simulink library "block_library"  (R2021b)
settings: Solver=VariableStepAuto  StartTime=0.0  StopTime=10.0  RelTol=1e-3
values from neighbouring files (symbols this model uses):
  d = param(17)    [get_full_state.m]
  gravity = [param(6), param(7),param(8)]    [get_ac_forces_moments.m]
  k_line = param(18)    [get_full_state.m]
  q = 0.5*rho*V_a^2    [aircraft_sizing_optimization.m]    (also in get_ac_forces_moments.m = state(11))
  r = state(12)    [get_ac_forces_moments.m]
  rho = rho_0*exp(-h/h1)    [aircraft_sizing_optimization.m]    (also in get_ac_forces_moments.m = param(2); get_simple_state.m = const(7))
undefined symbols (not defined in the file or in its folder): c, F, InitTheta, InitThetaDot, k_damp, k_pitch, k_roll, Light, magnitude, MIL, moi, motor_kt, motor_moi, state1, WindVelocity
libraries: aerolibwind2 x3, aerolibasang x2, vrlib x2, shared6dof x1, sharedtransform x1, sharedutil x1
settings Model: Creator=austm  LastModifiedBy=austm

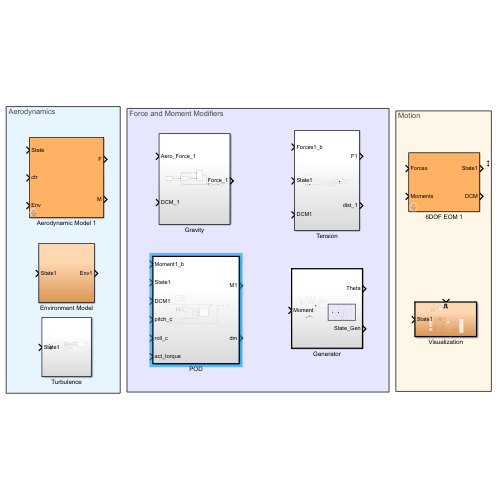
[thumbnail: Simulink's stored preview of the top-level diagram]
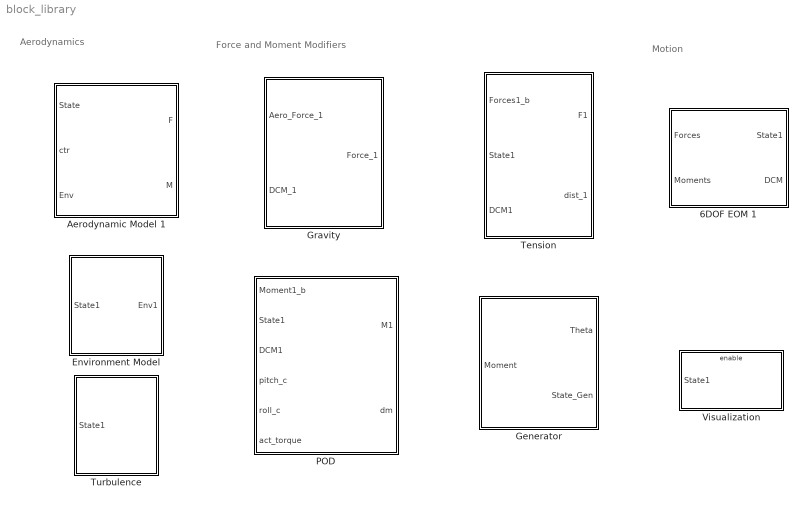
== system block_library ==
  note: Motion
  note: Force and Moment Modifiers
  note: Aerodynamics
  6DOF EOM 1 : Subsystem  VariantControl=eom3DOF  mask{XYZ=[0, 0, 0], uvw=[0, 0, 0], rpy=[0, 0, 0], pqr=[0, 0, 0], m=1, I=[1, 0, 0; 0, 1, 0; 0, 0, 1]}
      mask prompts: XYZ "Initial position in inertial axes [Xe,Ye,Ze]"; uvw "Initial velocity in body axes [U,v,w]"; rpy "Initial Euler orientation [roll, pitch, yaw]"; pqr "Initial body rotation rates [p,q,r]"; m "Initial mass"; I "Inertia"
  Aerodynamic Model 1 : Subsystem  VariantControl=aeroCONST  mask{CG=[0, 0, 0], CP=[0, 0, 0]}
      mask prompts: CG "Center of Gravity"; CP "Center of Pressure"
  Environment Model : Subsystem  VariantControl=aeroCONST
  Generator : Subsystem  TreatAsAtomicUnit=on
  Gravity : Subsystem
  POD : Subsystem  TreatAsAtomicUnit=on
  Tension : Subsystem
  Turbulence : Subsystem
  Visualization : Subsystem

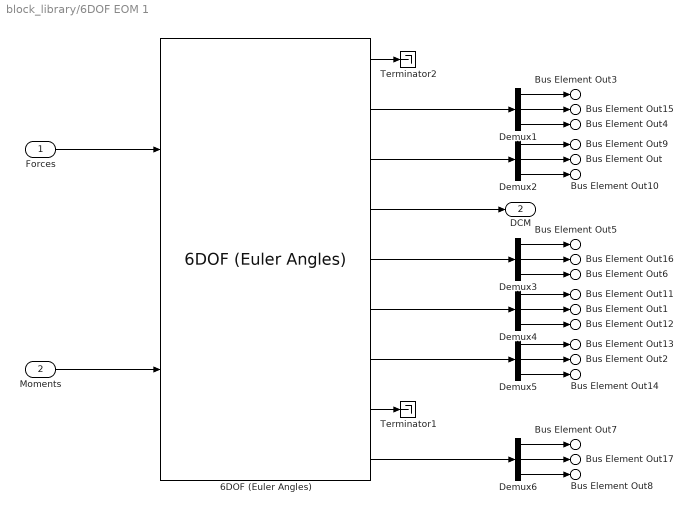
== system block_library/6DOF EOM 1 ==
  Forces : Inport
  Moments : Inport  Port=2
  6DOF (Euler Angles) : shared6dof/6DOF (Euler Angles)  units=Metric (MKS)  mtype=Fixed  rep=Euler Angles  xme_0=XYZ  Vm_0=uvw  eul_0=rpy  pm_0=pqr  mass_0=m  mass_e=0.5  mass_f=2.0  inertia=I  inertia_e=eye(3)  inertia_f=2*eye(3)  k_quat=1.0  vre_flag=on  abi_flag=on  aMode=0  xme_statename={'Xe', 'Ye', 'Ze'}  Vm_statename={'U', 'V', 'W'}  eul_statename={'phi', 'theta', 'psi'}  quat_statename={'qr', 'qi', 'qj','qk'}  pm_statename={'p', 'q', 'r'}  mass_statename=''
      settings: SourceProductBaseCode=AE,PW,DR,MT,UV,VE
  Demux{1..6} (6 alike) : Demux  Outputs=3
  Terminator1 : Terminator
  Terminator2 : Terminator
  Bus Element Out3 : Outport  VectorParamsAs1DForOutWhenUnconnected=off  PortName=State1  Element=Xe
  Bus Element Out4 : Outport  VectorParamsAs1DForOutWhenUnconnected=off  PortName=State1  Element=Ze
  Bus Element Out : Outport  VectorParamsAs1DForOutWhenUnconnected=off  PortName=State1  Element=theta
  Bus Element Out5 : Outport  VectorParamsAs1DForOutWhenUnconnected=off  PortName=State1  Element=u
  Bus Element Out6 : Outport  VectorParamsAs1DForOutWhenUnconnected=off  PortName=State1  Element=w
  Bus Element Out1 : Outport  VectorParamsAs1DForOutWhenUnconnected=off  PortName=State1  Element=q
  Bus Element Out2 : Outport  VectorParamsAs1DForOutWhenUnconnected=off  PortName=State1  Element=q_dot
  Bus Element Out7 : Outport  VectorParamsAs1DForOutWhenUnconnected=off  PortName=State1  Element=Axe
  Bus Element Out8 : Outport  VectorParamsAs1DForOutWhenUnconnected=off  PortName=State1  Element=Aze
  Bus Element Out15 : Outport  VectorParamsAs1DForOutWhenUnconnected=off  PortName=State1  Element=Ye
  Bus Element Out9 : Outport  VectorParamsAs1DForOutWhenUnconnected=off  PortName=State1  Element=phi
  Bus Element Out10 : Outport  VectorParamsAs1DForOutWhenUnconnected=off  PortName=State1  Element=psi
  Bus Element Out16 : Outport  VectorParamsAs1DForOutWhenUnconnected=off  PortName=State1  Element=v
  Bus Element Out11 : Outport  VectorParamsAs1DForOutWhenUnconnected=off  PortName=State1  Element=p
  Bus Element Out12 : Outport  VectorParamsAs1DForOutWhenUnconnected=off  PortName=State1  Element=r
  Bus Element Out13 : Outport  VectorParamsAs1DForOutWhenUnconnected=off  PortName=State1  Element=p_dot
  Bus Element Out14 : Outport  VectorParamsAs1DForOutWhenUnconnected=off  PortName=State1  Element=r_dot
  Bus Element Out17 : Outport  VectorParamsAs1DForOutWhenUnconnected=off  PortName=State1  Element=Aye
  DCM : Outport  Port=2
  wires:
  6DOF (Euler Angles)/2 -> Demux1/1
  6DOF (Euler Angles)/4 -> DCM/1
  6DOF (Euler Angles)/1 -> Terminator2/1
  Demux6/2 -> Bus Element Out17/1
  Demux6/3 -> Bus Element Out8/1
  Demux6/1 -> Bus Element Out7/1
  6DOF (Euler Angles)/9 -> Demux6/1
  6DOF (Euler Angles)/7 -> Demux5/1
  Demux5/3 -> Bus Element Out14/1
  Demux5/2 -> Bus Element Out2/1
  Demux5/1 -> Bus Element Out13/1
  6DOF (Euler Angles)/6 -> Demux4/1
  Demux4/3 -> Bus Element Out12/1
  Demux4/2 -> Bus Element Out1/1
  Demux4/1 -> Bus Element Out11/1
  Demux3/3 -> Bus Element Out6/1
  Demux3/2 -> Bus Element Out16/1
  Demux3/1 -> Bus Element Out5/1
  6DOF (Euler Angles)/5 -> Demux3/1
  Demux2/3 -> Bus Element Out10/1
  Demux2/2 -> Bus Element Out/1
  Demux2/1 -> Bus Element Out9/1
  Demux1/1 -> Bus Element Out3/1
  Demux1/3 -> Bus Element Out4/1
  Demux1/2 -> Bus Element Out15/1
  6DOF (Euler Angles)/3 -> Demux2/1
  Moments/1 -> 6DOF (Euler Angles)/2
  Forces/1 -> 6DOF (Euler Angles)/1
  6DOF (Euler Angles)/8 -> Terminator1/1

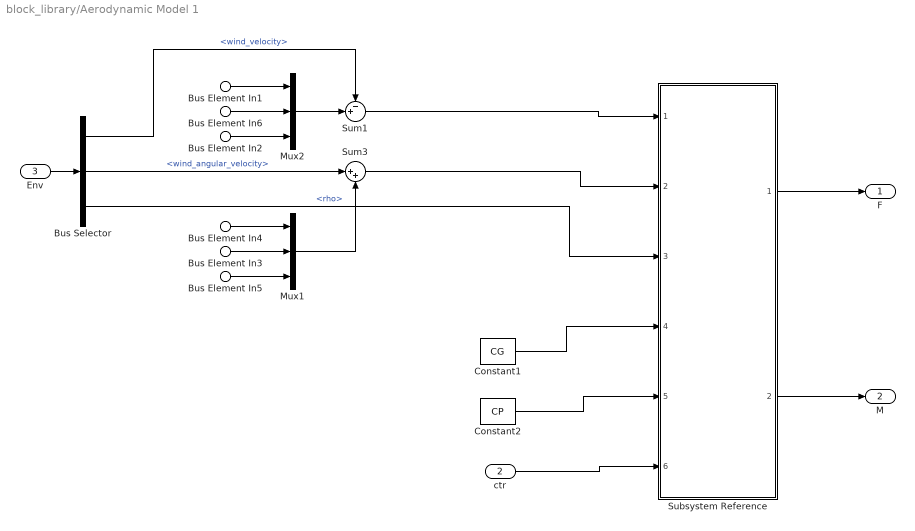
== system block_library/Aerodynamic Model 1 ==
  Bus Element In1 : Inport  PortName=State  Element=u
  Bus Element In2 : Inport  PortName=State  Element=w
  Bus Element In3 : Inport  PortName=State  Element=q
  Bus Element In6 : Inport  PortName=State  Element=v
  Bus Element In4 : Inport  PortName=State  Element=p
  Bus Element In5 : Inport  PortName=State  Element=r
  ctr : Inport  Port=2
  Env : Inport  Port=3
  Bus Selector : BusSelector  OutputSignals=wind_velocity,wind_angular_velocity,rho
  Constant1 : Constant  Value=CG
  Constant2 : Constant  Value=CP
  Mux1 : Mux  Inputs=3
  Mux2 : Mux  Inputs=3
  Subsystem Reference : Subsystem  ReferencedSubsystem=Aerodynamics
  Sum1 : Sum  Inputs=-+|  InputSameDT=on  SaturateOnIntegerOverflow=on  OutDataTypeStr=Inherit: Same as first input
  Sum3 : Sum  Inputs=|++  InputSameDT=on  SaturateOnIntegerOverflow=on  OutDataTypeStr=Inherit: Same as first input
  F : Outport  Unit=N  VectorParamsAs1DForOutWhenUnconnected=off
  M : Outport  Port=2  Unit=N*m  VectorParamsAs1DForOutWhenUnconnected=off
  wires:
  Bus Selector/1 -> Sum1/1  "<wind_velocity>"
  Mux2/1 -> Sum1/2
  Mux1/1 -> Sum3/2
  Bus Selector/2 -> Sum3/1  "<wind_angular_velocity>"
  Bus Element In5/1 -> Mux1/3
  Bus Element In3/1 -> Mux1/2
  Bus Element In4/1 -> Mux1/1
  Bus Element In1/1 -> Mux2/1
  Bus Element In6/1 -> Mux2/2
  Bus Element In2/1 -> Mux2/3
  Sum1/1 -> Subsystem Reference/1
  Sum3/1 -> Subsystem Reference/2
  Bus Selector/3 -> Subsystem Reference/3  "<rho>"
  Constant1/1 -> Subsystem Reference/4
  Constant2/1 -> Subsystem Reference/5
  Subsystem Reference/1 -> F/1
  Subsystem Reference/2 -> M/1
  ctr/1 -> Subsystem Reference/6
  Env/1 -> Bus Selector/1

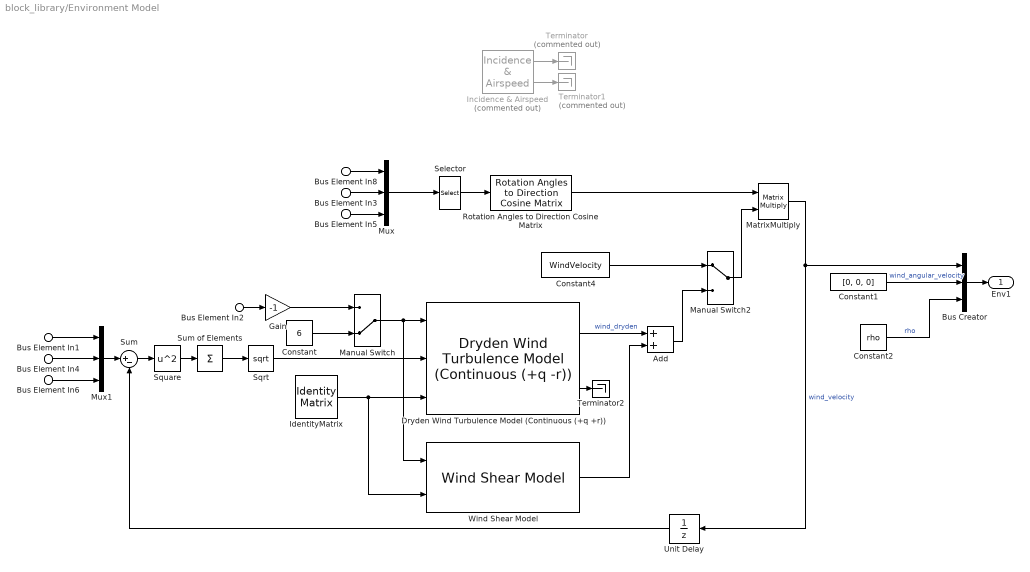
== system block_library/Environment Model ==
  Bus Element In3 : Inport  PortName=State1  Element=theta
  Bus Element In8 : Inport  PortName=State1  Element=phi
  Bus Element In5 : Inport  PortName=State1  Element=psi
  Bus Element In1 : Inport  PortName=State1  Element=u
  Bus Element In2 : Inport  PortName=State1  Element=Ze
  Bus Element In4 : Inport  PortName=State1  Element=v
  Bus Element In6 : Inport  PortName=State1  Element=w
  Add : Sum
  Bus Creator : BusCreator  Inputs=3
  Constant : Constant  Value=6
  Constant1 : Constant  Value=[0, 0, 0]
  Constant2 : Constant  Value=rho
  Constant4 : Constant  Value=WindVelocity
  Dryden Wind Turbulence Model (Continuous (+q +r)) : aerolibwind2/Dryden Wind Turbulence Model  (Continuous (+q -r))  units=Metric (MKS)  spec=MIL-F-8785C  model=Continuous Dryden (+q +r)  W20=WindVelocity(1)  Wdeg=0  TurbProb=10^-2 - Light  L_high=533.4  Wingspan=3  ts=0.1  Seed=[23341 23342 23343 23344]  T_on=on
  Gain : Gain  Gain=-1
  IdentityMatrix : IdentityMatrix  OutputDimensions=3
  Incidence & Airspeed : aerolibasang/Incidence  & Airspeed  Commented=on
      settings: SourceProductBaseCode=AE
  Manual Switch : ManualSwitch  CurrentSetting=0
  Manual Switch2 : ManualSwitch
  MatrixMultiply : Product  Multiplication=Matrix(*)
  Mux : Mux  Inputs=3
  Mux1 : Mux  Inputs=3
  Rotation Angles to Direction Cosine Matrix : sharedtransform/Rotation Angles to Direction Cosine Matrix  rotationOrder=ZYX  aMode=aMode
      settings: SourceProductBaseCode=AE,PW,DR,MT,UV,VE
  Selector : Selector  InputPortWidth=3  IndexOptions=Index vector (dialog)  Indices=[3 2 1]  OutputSizes=1
  Sqrt : Sqrt  SaturateOnIntegerOverflow=on
  Square : Math  Operator=square  SaturateOnIntegerOverflow=on
  Sum : Sum  Inputs=|+-
  Sum of Elements : Sum  Inputs=+
  Terminator : Terminator  Commented=on
  Terminator1 : Terminator  Commented=on
  Terminator2 : Terminator
  Unit Delay : UnitDelay  InitialCondition=norm(WindVelocity)  SampleTime=-1  HasFrameUpgradeWarning=on
  Wind Shear Model : aerolibwind2/Wind Shear Model  units=Metric (MKS)  phase=Category C - Terminal Flight Phase  W_20=norm(WindVelocity)  Wdeg=atan2d(WindVelocity(2), WindVelocity(1))+180
  Env1 : Outport
  wires:
  Constant1/1 -> Bus Creator/2  "wind_angular_velocity"
  Dryden Wind Turbulence Model (Continuous (+q +r))/1 -> Add/1  "wind_dryden"
  Rotation Angles to Direction Cosine Matrix/1 -> MatrixMultiply/1
  Bus Element In5/1 -> Mux/3
  Mux/1 -> Selector/1
  Incidence & Airspeed/2 -> Terminator1/1
  Incidence & Airspeed/1 -> Terminator/1
  Constant2/1 -> Bus Creator/3  "rho"
  Bus Element In8/1 -> Mux/1
  Bus Element In3/1 -> Mux/2
  MatrixMultiply/1 -> Bus Creator/1, Unit Delay/1  "wind_velocity"
  Selector/1 -> Rotation Angles to Direction Cosine Matrix/1
  Bus Creator/1 -> Env1/1
  Manual Switch/1 -> Dryden Wind Turbulence Model (Continuous (+q +r))/1, Wind Shear Model/1
  Bus Element In1/1 -> Mux1/1
  IdentityMatrix/1 -> Wind Shear Model/2, Dryden Wind Turbulence Model (Continuous (+q +r))/3
  Dryden Wind Turbulence Model (Continuous (+q +r))/2 -> Terminator2/1
  Add/1 -> Manual Switch2/2
  Bus Element In2/1 -> Gain/1
  Bus Element In4/1 -> Mux1/2
  Bus Element In6/1 -> Mux1/3
  Mux1/1 -> Sum/1
  Sum/1 -> Square/1
  Square/1 -> Sum of Elements/1
  Sum of Elements/1 -> Sqrt/1
  Sqrt/1 -> Dryden Wind Turbulence Model (Continuous (+q +r))/2
  Constant/1 -> Manual Switch/2
  Gain/1 -> Manual Switch/1
  Unit Delay/1 -> Sum/2
  Wind Shear Model/1 -> Add/2
  Constant4/1 -> Manual Switch2/1
  Manual Switch2/1 -> MatrixMultiply/2

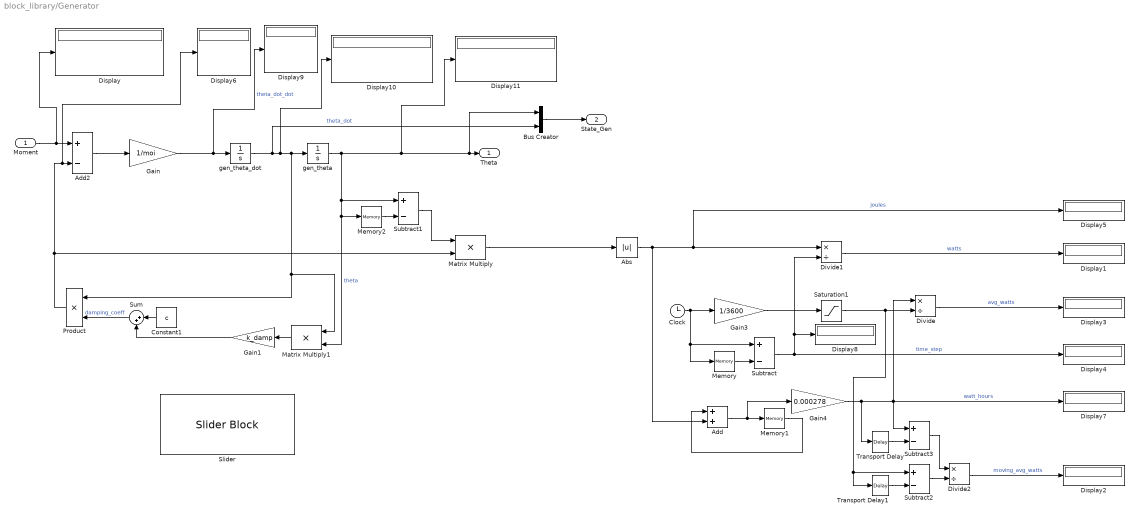
== system block_library/Generator ==
  Moment : Inport
  Abs : Abs
  Add : Sum
  Add2 : Sum  Inputs=+-
  Bus Creator : BusCreator  Inputs=2
  Clock : Clock
  Constant1 : Constant  Value=c
  Display{,1..11} (12 alike) : Display
      Display settings: Format=long_e  Decimation=6
      Display10 settings: Format=long_e
      Display11 settings: Format=long_e
  Divide : Product  Inputs=*/
  Divide1 : Product  Inputs=*/
  Divide2 : Product  Inputs=*/
  Gain : Gain  Gain=1/moi
  Gain1 : Gain  Gain=k_damp
  Gain3 : Gain  Gain=1/3600
  Gain4 : Gain  Gain=0.000278
  Matrix Multiply : Product
  Matrix Multiply1 : Product
  Memory : Memory  InitialCondition=-.001
  Memory1 : Memory
  Memory2 : Memory
  Product : Product
  Saturation1 : Saturate  UpperLimit=inf  LowerLimit=0.00001
  Slider : SliderBlock  ScaleMax=500
  Subtract{,1..3} (4 alike) : Sum  Inputs=+-
  Sum : Sum  Inputs=|++
  Transport Delay : TransportDelay  DelayTime=30  BufferSize=10240
  Transport Delay1 : TransportDelay  DelayTime=30  BufferSize=10240
  gen_theta : Integrator  InitialCondition=InitTheta
  gen_theta_dot : Integrator  InitialCondition=InitThetaDot
  Theta : Outport
  State_Gen : Outport  Port=2
  wires:
  Bus Creator/1 -> State_Gen/1
  Saturation1/1 -> Transport Delay1/1, Subtract2/1, Divide/2
  Divide2/1 -> Display2/1  "moving_avg_watts"
  Subtract3/1 -> Divide2/1
  Transport Delay/1 -> Subtract3/2
  Subtract2/1 -> Divide2/2
  Transport Delay1/1 -> Subtract2/2
  Gain1/1 -> Sum/2
  Sum/1 -> Product/2  "damping_coeff"
  Constant1/1 -> Sum/1
  Memory2/1 -> Subtract1/2
  Gain4/1 -> Transport Delay/1, Divide/1, Subtract3/1, Display7/1  "watt_hours"
  Memory1/1 -> Add/1
  Add/1 -> Gain4/1, Memory1/1
  Matrix Multiply/1 -> Abs/1
  Divide1/1 -> Display1/1  "watts"
  Subtract/1 -> Display4/1, Display8/1, Divide1/2  "time_step"
  Memory/1 -> Subtract/2
  Divide/1 -> Display3/1  "avg_watts"
  Gain3/1 -> Saturation1/1
  Clock/1 -> Gain3/1, Subtract/1, Memory/1
  Product/1 -> Display6/1, Add2/2, Matrix Multiply/2
  Matrix Multiply1/1 -> Gain1/1
  Abs/1 -> Add/2, Divide1/1, Display5/1  "joules"
  Subtract1/1 -> Matrix Multiply/1
  gen_theta/1 -> Subtract1/1, Memory2/1, Matrix Multiply1/2, Display11/1, Bus Creator/1, Theta/1  "theta"
  gen_theta_dot/1 -> Display10/1, gen_theta/1, Matrix Multiply1/1, Product/1, Bus Creator/2  "theta_dot"
  Gain/1 -> Display9/1, gen_theta_dot/1  "theta_dot_dot"
  Add2/1 -> Gain/1
  Moment/1 -> Add2/1, Display/1

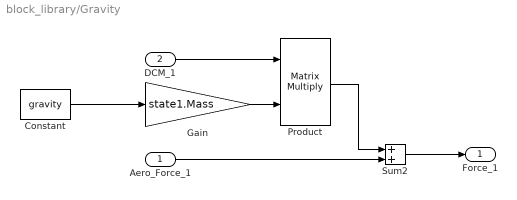
== system block_library/Gravity ==
  Aero_Force_1 : Inport
  DCM_1 : Inport  Port=2
  Constant : Constant  Value=gravity
  Gain : Gain  Gain=state1.Mass
  Product : Product  Multiplication=Matrix(*)
  Sum2 : Sum  InputSameDT=on  SaturateOnIntegerOverflow=on  OutDataTypeStr=Inherit: Same as first input
  Force_1 : Outport
  wires:
  Gain/1 -> Product/2
  Product/1 -> Sum2/1
  DCM_1/1 -> Product/1
  Aero_Force_1/1 -> Sum2/2
  Sum2/1 -> Force_1/1
  Constant/1 -> Gain/1

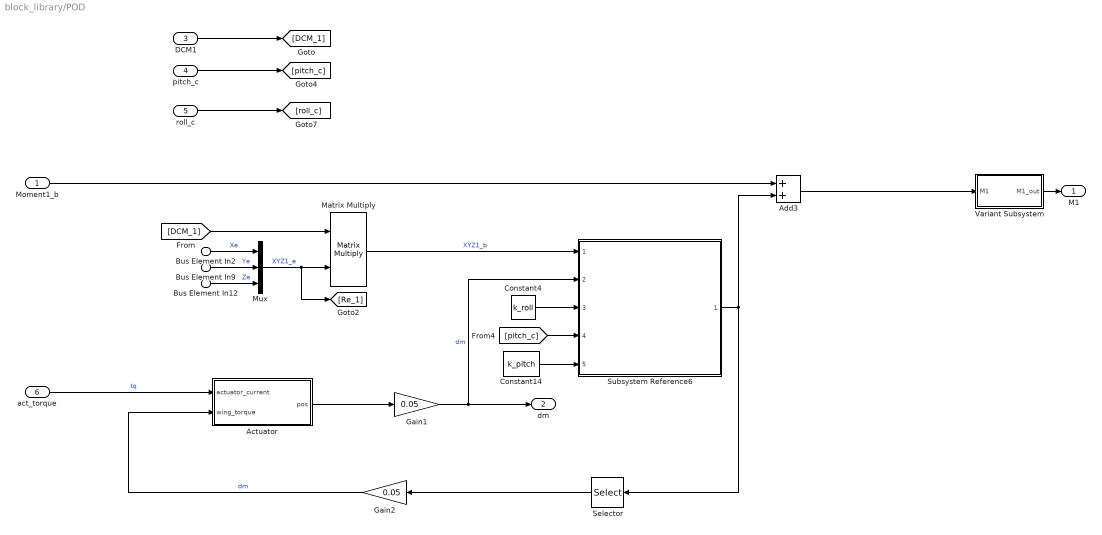
== system block_library/POD ==
  Moment1_b : Inport
  Bus Element In12 : Inport  Port=2  PortName=State1  Element=Ze
  Bus Element In2 : Inport  Port=2  PortName=State1  Element=Xe
  Bus Element In9 : Inport  Port=2  PortName=State1  Element=Ye
  DCM1 : Inport  Port=3
  pitch_c : Inport  Port=4
  roll_c : Inport  Port=5
  act_torque : Inport  Port=6
  Actuator : Subsystem
  Add3 : Sum
  Constant14 : Constant  Value=k_pitch
  Constant4 : Constant  Value=k_roll
  Gain1 : Gain  Gain=0.05
  Gain2 : Gain  Gain=0.05
  Matrix Multiply : Product  Multiplication=Matrix(*)
  Mux : Mux  Inputs=3
  Selector : Selector  InputPortWidth=3  IndexOptions=Index vector (dialog)  Indices=1  OutputSizes=1
  Subsystem Reference6 : Subsystem  ReferencedSubsystem=control_moments
  Variant Subsystem : Subsystem  Variant=on
  M1 : Outport
  dm : Outport  Port=2
  wires:
  Constant14/1 -> Subsystem Reference6/5
  [pitch_c] -> Subsystem Reference6/4
  Constant4/1 -> Subsystem Reference6/3
  Subsystem Reference6/1 -> Add3/2, Selector/1
  Matrix Multiply/1 -> Subsystem Reference6/1  "XYZ1_b"
  Moment1_b/1 -> Add3/1
  DCM1/1 -> [DCM_1]
  Bus Element In2/1 -> Mux/1  "Xe"
  Bus Element In12/1 -> Mux/3  "Ze"
  Bus Element In9/1 -> Mux/2  "Ye"
  Mux/1 -> Matrix Multiply/2, [Re_1]  "XYZ1_e"
  [DCM_1] -> Matrix Multiply/1
  Variant Subsystem/1(M1_out) -> M1/1
  roll_c/1 -> [roll_c]
  pitch_c/1 -> [pitch_c]
  Add3/1 -> Variant Subsystem/1(M1)
  Gain1/1 -> Subsystem Reference6/2, dm/1  "dm"
  act_torque/1 -> Actuator/1(actuator_current)  "tq"
  Selector/1 -> Gain2/1
  Actuator/1(pos) -> Gain1/1
  Gain2/1 -> Actuator/2(wing_torque)  "dm"

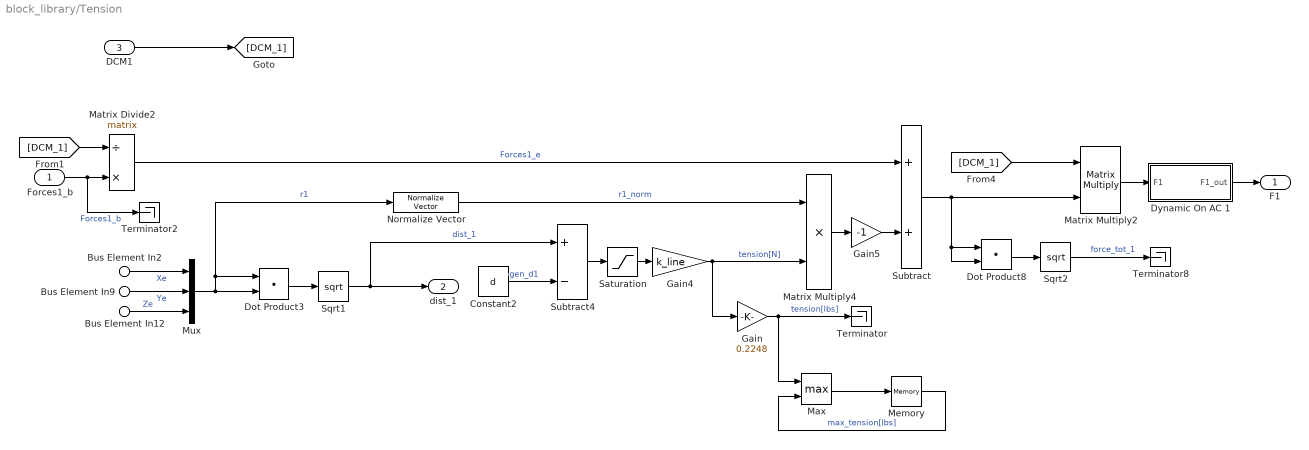
== system block_library/Tension ==
  Forces1_b : Inport
  Bus Element In12 : Inport  Port=2  PortName=State1  Element=Ze
  Bus Element In2 : Inport  Port=2  PortName=State1  Element=Xe
  Bus Element In9 : Inport  Port=2  PortName=State1  Element=Ye
  DCM1 : Inport  Port=3
  Constant2 : Constant  Value=d
  Dot Product3 : DotProduct  InputSameDT=on  OutDataTypeStr=Inherit: Inherit via internal rule
  Dot Product8 : DotProduct  InputSameDT=on  OutDataTypeStr=Inherit: Inherit via internal rule
  Dynamic On AC 1 : Subsystem  Variant=on
  Gain : Gain  Gain=0.2248
  Gain4 : Gain  Gain=k_line
  Gain5 : Gain  Gain=-1
  Matrix Divide2 : Product  Inputs=/*  Multiplication=Matrix(*)
  Matrix Multiply2 : Product  Multiplication=Matrix(*)
  Matrix Multiply4 : Product
  Max : MinMax  Function=max  Inputs=2
  Memory : Memory
  Mux : Mux  Inputs=3
  Normalize Vector : vrlib/Utilities/Normalize Vector  maxzero=0
  Saturation : Saturate  UpperLimit=inf  LowerLimit=0
  Sqrt1 : Sqrt  SaturateOnIntegerOverflow=on
  Sqrt2 : Sqrt  SaturateOnIntegerOverflow=on
  Subtract : Sum
  Subtract4 : Sum  Inputs=+-
  Terminator : Terminator
  Terminator2 : Terminator
  Terminator8 : Terminator
  F1 : Outport  Unit=N  VectorParamsAs1DForOutWhenUnconnected=off
  dist_1 : Outport  Port=2
  wires:
  Bus Element In2/1 -> Mux/1  "Xe"
  Bus Element In9/1 -> Mux/2  "Ye"
  Bus Element In12/1 -> Mux/3  "Ze"
  DCM1/1 -> [DCM_1]
  [DCM_1] -> Matrix Divide2/1
  Matrix Multiply2/1 -> Dynamic On AC 1/1(F1)
  [DCM_1] -> Matrix Multiply2/1
  Forces1_b/1 -> Terminator2/1, Matrix Divide2/2  "Forces1_b"
  Subtract/1 -> Dot Product8/2, Dot Product8/1, Matrix Multiply2/2
  Mux/1 -> Normalize Vector/1, Dot Product3/1, Dot Product3/2  "r1"
  Dot Product3/1 -> Sqrt1/1
  Sqrt1/1 -> Subtract4/1, dist_1/1  "dist_1"
  Gain5/1 -> Subtract/2
  Dynamic On AC 1/1(F1_out) -> F1/1
  Matrix Divide2/1 -> Subtract/1  "Forces1_e"
  Sqrt2/1 -> Terminator8/1  "force_tot_1"
  Dot Product8/1 -> Sqrt2/1
  Normalize Vector/1 -> Matrix Multiply4/1  "r1_norm"
  Gain4/1 -> Gain/1, Matrix Multiply4/2  "tension[N]"
  Constant2/1 -> Subtract4/2  "gen_d1"
  Matrix Multiply4/1 -> Gain5/1
  Subtract4/1 -> Saturation/1
  Saturation/1 -> Gain4/1
  Gain/1 -> Max/1, Terminator/1  "tension[lbs]"
  Max/1 -> Memory/1
  Memory/1 -> Max/2  "max_tension[lbs]"

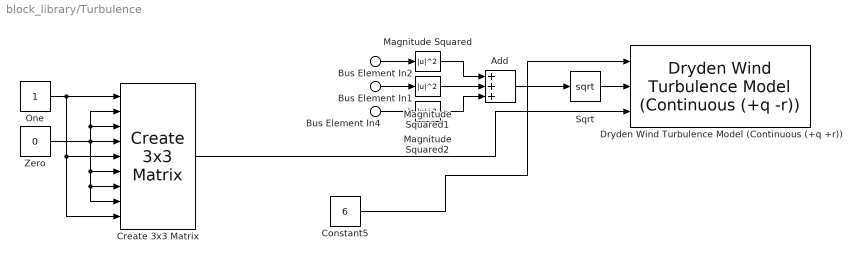
== system block_library/Turbulence ==
  Bus Element In2 : Inport  PortName=State1  Element=u
  Bus Element In1 : Inport  PortName=State1  Element=v
  Bus Element In4 : Inport  PortName=State1  Element=w
  Add : Sum  Inputs=+++
  Constant5 : Constant  Value=6
  Create 3x3 Matrix : sharedutil/Create 3x3 Matrix  aMode=aMode
      settings: SourceProductBaseCode=AE,PW,DR,MT,UV,VE
  Dryden Wind Turbulence Model (Continuous (+q +r)) : aerolibwind2/Dryden Wind Turbulence Model  (Continuous (+q -r))  units=Metric (MKS)  spec=MIL-F-8785C  model=Continuous Dryden (+q +r)  W20=3  Wdeg=180  TurbProb=10^-2 - Light  L_high=533.4  Wingspan=3  ts=0.1  Seed=[23341 23342 23343 23344]  T_on=off
  Magnitude Squared : Math  Operator=magnitude^2  SaturateOnIntegerOverflow=on
  Magnitude Squared1 : Math  Operator=magnitude^2  SaturateOnIntegerOverflow=on
  Magnitude Squared2 : Math  Operator=magnitude^2  SaturateOnIntegerOverflow=on
  One : Constant  OutDataTypeStr=Inherit: Inherit via back propagation
  Sqrt : Sqrt  SaturateOnIntegerOverflow=on
  Zero : Constant  Value=0  OutDataTypeStr=Inherit: Inherit via back propagation
  wires:
  Magnitude Squared2/1 -> Add/3
  Magnitude Squared/1 -> Add/1
  Constant5/1 -> Dryden Wind Turbulence Model (Continuous (+q +r))/1
  Magnitude Squared1/1 -> Add/2
  Zero/1 -> Create 3x3 Matrix/8, Create 3x3 Matrix/7, Create 3x3 Matrix/6, Create 3x3 Matrix/3, Create 3x3 Matrix/2, Create 3x3 Matrix/4
  Bus Element In4/1 -> Magnitude Squared2/1
  Bus Element In2/1 -> Magnitude Squared/1
  One/1 -> Create 3x3 Matrix/9, Create 3x3 Matrix/5, Create 3x3 Matrix/1
  Sqrt/1 -> Dryden Wind Turbulence Model (Continuous (+q +r))/2
  Add/1 -> Sqrt/1
  Bus Element In1/1 -> Magnitude Squared1/1
  Create 3x3 Matrix/1 -> Dryden Wind Turbulence Model (Continuous (+q +r))/3

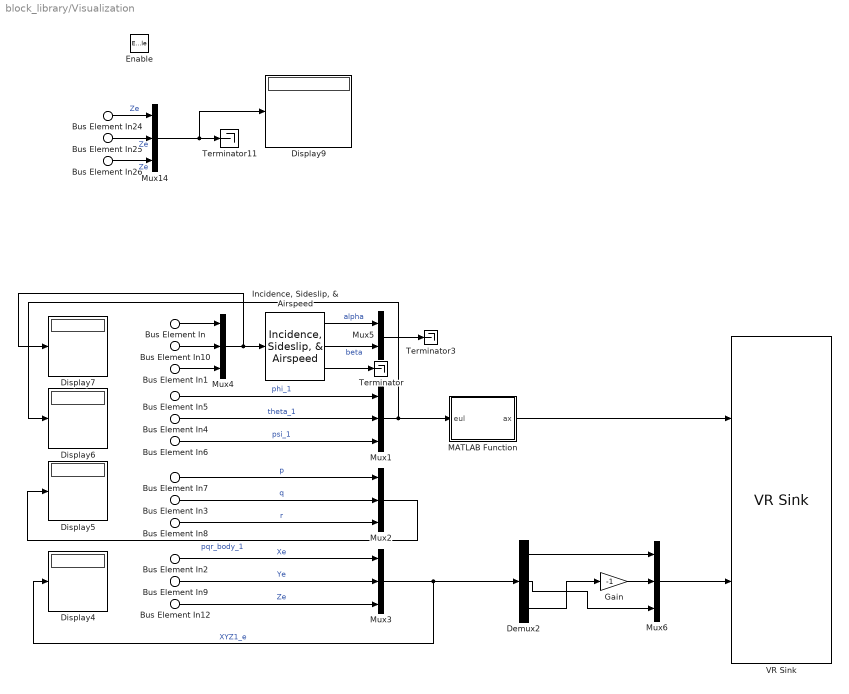
== system block_library/Visualization ==
  Bus Element In : Inport  PortName=State1  Element=u
  Bus Element In1 : Inport  PortName=State1  Element=w
  Bus Element In3 : Inport  PortName=State1  Element=q
  Bus Element In4 : Inport  PortName=State1  Element=theta
  Bus Element In12 : Inport  PortName=State1  Element=Ze
  Bus Element In2 : Inport  PortName=State1  Element=Xe
  Bus Element In10 : Inport  PortName=State1  Element=v
  Bus Element In5 : Inport  PortName=State1  Element=phi
  Bus Element In6 : Inport  PortName=State1  Element=psi
  Bus Element In7 : Inport  PortName=State1  Element=p
  Bus Element In8 : Inport  PortName=State1  Element=r
  Bus Element In9 : Inport  PortName=State1  Element=Ye
  Bus Element In24 : Inport  PortName=State1  Element=Axe
  Bus Element In25 : Inport  PortName=State1  Element=Aye
  Bus Element In26 : Inport  PortName=State1  Element=Aze
  Enable : EnablePort
  Demux2 : Demux  Outputs=3
  Display{4..7,9} (5 alike) : Display
  Gain : Gain  Gain=-1
  "Incidence, Sideslip, & Airspeed" : aerolibasang/Incidence, Sideslip, & Airspeed
  MATLAB Function : MATLAB Function  TreatAsAtomicUnit=on
  Mux{1..4,6,14} (6 alike) : Mux  Inputs=3
  Mux5 : Mux  Inputs=2
  Terminator : Terminator
  Terminator11 : Terminator
  Terminator3 : Terminator
  VR Sink : vrlib/VR Sink  InstantiateOnLoad=on  SampleTime=0.05  ViewEnable=on  RemoteChange=off  RemoteView=off  FieldsWritten=aircraft_1.rotation.4.1.1.double#aircraft_1.translation.3.1.1.double  WorldFileName=aero_gen_virtual_environment.wrl  AutoView=off  VideoDimensions=[]  AllowVariableSize=off
  wires:
  Mux3/1 -> Display4/1, Demux2/1  "XYZ1_e"
  Bus Element In2/1 -> Mux3/1  "Xe"
  Bus Element In12/1 -> Mux3/3  "Ze"
  Mux2/1 -> Display5/1  "pqr_body_1"
  "Incidence, Sideslip, & Airspeed"/2 -> Mux5/2  "beta"
  "Incidence, Sideslip, & Airspeed"/1 -> Mux5/1  "alpha"
  Mux4/1 -> Display7/1, "Incidence, Sideslip, & Airspeed"/1
  Bus Element In10/1 -> Mux4/2
  Bus Element In8/1 -> Mux2/3  "r"
  Bus Element In7/1 -> Mux2/1  "p"
  Bus Element In6/1 -> Mux1/3  "psi_1"
  Bus Element In5/1 -> Mux1/1  "phi_1"
  Bus Element In4/1 -> Mux1/2  "theta_1"
  Bus Element In3/1 -> Mux2/2  "q"
  Bus Element In1/1 -> Mux4/3
  "Incidence, Sideslip, & Airspeed"/3 -> Terminator/1
  Bus Element In9/1 -> Mux3/2  "Ye"
  Demux2/1 -> Mux6/1
  Demux2/3 -> Gain/1
  Gain/1 -> Mux6/2
  Demux2/2 -> Mux6/3
  Bus Element In/1 -> Mux4/1
  Mux14/1 -> Display9/1, Terminator11/1
  Bus Element In25/1 -> Mux14/2  "Ze"
  Bus Element In26/1 -> Mux14/3  "Ze"
  Bus Element In24/1 -> Mux14/1  "Ze"
  Mux1/1 -> Display6/1, MATLAB Function/1(eul)
  Mux5/1 -> Terminator3/1
  MATLAB Function/1(ax) -> VR Sink/1
  Mux6/1 -> VR Sink/2

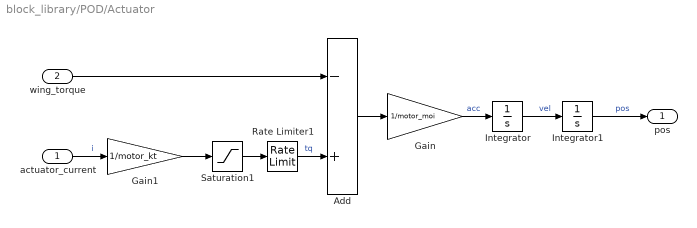
== system block_library/POD/Actuator ==
  actuator_current : Inport
  wing_torque : Inport  Port=2
  Add : Sum  Inputs=-+
  Gain : Gain  Gain=1/motor_moi
  Gain1 : Gain  Gain=1/motor_kt
  Integrator : Integrator  UpperSaturationLimit=100  LowerSaturationLimit=-100
  Integrator1 : Integrator  UpperSaturationLimit=80  LowerSaturationLimit=-80
  Rate Limiter1 : RateLimiter  RisingSlewLimit=inf  FallingSlewLimit=-inf  SampleTimeMode=inherited
  Saturation1 : Saturate  UpperLimit=inf  LowerLimit=-inf
  pos : Outport
  wires:
  Integrator/1 -> Integrator1/1  "vel"
  Gain/1 -> Integrator/1  "acc"
  Add/1 -> Gain/1
  Integrator1/1 -> pos/1  "pos"
  actuator_current/1 -> Gain1/1  "i"
  Saturation1/1 -> Rate Limiter1/1
  wing_torque/1 -> Add/1
  Gain1/1 -> Saturation1/1
  Rate Limiter1/1 -> Add/2  "tq"

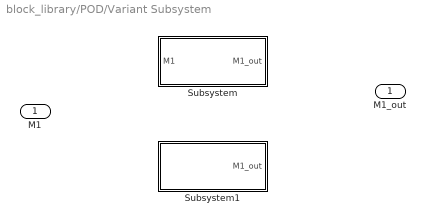
== system block_library/POD/Variant Subsystem ==
  M1 : Inport
  Subsystem : Subsystem  VariantControl=ac1_moments > 0
  Subsystem1 : Subsystem  VariantControl="ac1_moments ==  0"
  M1_out : Outport

== system block_library/Tension/Dynamic On AC 1 ==
  F1 : Inport
  Subsystem : Subsystem  VariantControl=ac1_forces > 0
  Subsystem1 : Subsystem  VariantControl="ac1_forces ==  0"
  F1_out : Outport

== system block_library/POD/Variant Subsystem/Subsystem ==
  M1 : Inport
  M1_out : Outport
  wires:
  M1/1 -> M1_out/1

== system block_library/POD/Variant Subsystem/Subsystem1 ==
  Constant : Constant  Value=0
  Mux : Mux  Inputs=3
  M1_out : Outport
  wires:
  Mux/1 -> M1_out/1
  Constant/1 -> Mux/3, Mux/2, Mux/1

== system block_library/Tension/Dynamic On AC 1/Subsystem ==
  F1 : Inport
  F1_out : Outport
  wires:
  F1/1 -> F1_out/1

== system block_library/Tension/Dynamic On AC 1/Subsystem1 ==
  Constant : Constant  Value=0
  Mux : Mux  Inputs=3
  F1_out : Outport
  wires:
  Mux/1 -> F1_out/1
  Constant/1 -> Mux/3, Mux/2, Mux/1

== matlab function block_library/Visualization/MATLAB Function ==
  data: ax output; eul input
function ax = eul2ax(eul)
% c1 = cos(u(3)/2);
% c2 = cos(u(2)/2);
% c3 = cos(u(1)/2);
% s1 = sin(u(3)/2);
% s2 = sin(u(2)/2);
% s3 = sin(u(1)/2);

% q = eul2quat([-u(1), -u(3), u(2)]);
 eul = [eul(1), eul(2), -eul(3)];
 q = eul2quat(eul, 'XYZ');
 q = [q(1), q(2), q(4), q(3)];
axis_ang = quat2axang(q);
ax = axis_ang';


end
